simulink model "aae301_final_simulink"  (R2021a)
settings: Solver=VariableStepAuto  StartTime=0.0  StopTime=10.0  RelTol=1e-3
libraries: simulink x1
settings Model: Creator=cjobr  LastModifiedBy=cjobr

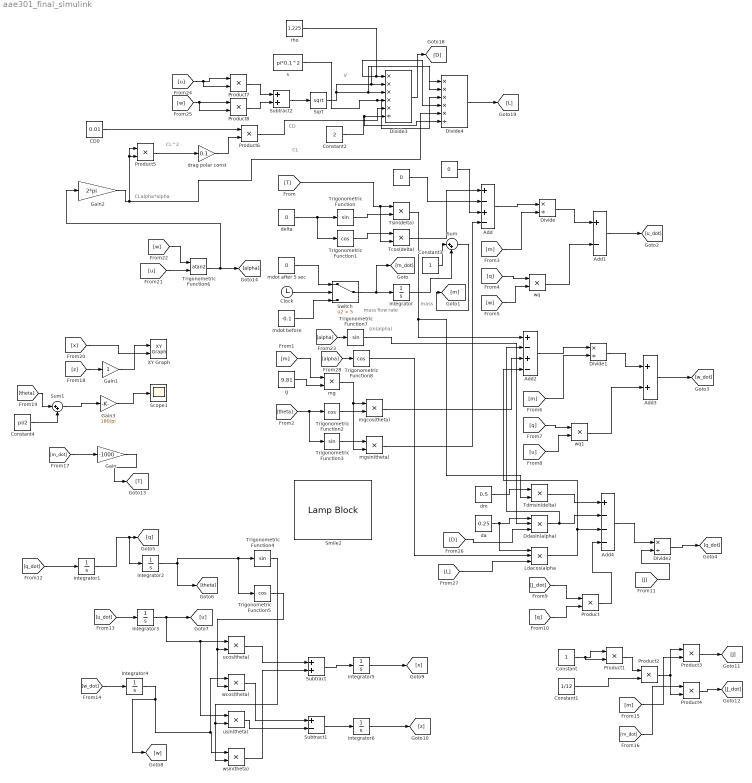
== system aae301_final_simulink ==
  note: V
  note: CL
  note: CD
  note: CL^2
  note: CLalpha*alpha
  note: sin(alpha)
  note: mass flow rate
  note: mass
  "  " : Constant  Value=0
  "    " : Constant  Value=0
  Add : Sum  Inputs=+-+-
  Add1 : Sum  Inputs=+-
  Add2 : Sum  Inputs=+-+-
  Add3 : Sum
  Add4 : Sum  Inputs=+---
  CD0 : Constant  Value=0.01
  Clock : Clock
  Constant : Constant
  Constant1 : Constant  Value=1/12
  Constant2 : Constant  Value=2
  Constant3 : Constant
  Constant4 : Constant  Value=pi/2
  Ddasin(alpha) : Product  Inputs=3
  Divide : Product  Inputs=*/
  Divide1 : Product  Inputs=*/
  Divide2 : Product  Inputs=*/
  Divide3 : Product  Inputs=*****/
  Divide4 : Product  Inputs=*****/
  Gain : Gain  Gain=-1000
  Gain1 : Gain
  Gain2 : Gain  Gain=2*pi
  Gain3 : Gain  Gain=180/pi
  Integrator{,1..6} (7 alike) : Integrator
  Ldacos(alpha : Product  Inputs=3
  Product{,1..8} (9 alike) : Product
  Scope1 : Scope
  Smile2 : LampBlock  LabelPosition=Hide  Icon=Smile2
  Sqrt : Sqrt  SaturateOnIntegerOverflow=on
  Subtract : Sum
  Subtract1 : Sum  Inputs=+-
  Subtract2 : Sum
  Sum : Sum  Inputs=|++
  Sum1 : Sum  Inputs=|++
  Switch : Switch  Criteria=u2 > Threshold  Threshold=5
  Tcos(delta) : Product
  Tdmsin(delta) : Product
  Trigonometric Function{,3..4,7} (4 alike) : Trigonometry
  Trigonometric Function{1..2,5,8} (4 alike) : Trigonometry  Operator=cos
  Trigonometric Function6 : Trigonometry  Operator=atan2
  Tsin(delta) : Product
  XY Graph : simulink/Sinks/XY Graph  xmin=-100  xmax=1700  ymin=-10  ymax=3300  st=9
  da : Constant  Value=0.25
  delta : Constant  Value=0
  dm : Constant  Value=0.5
  drag polar const : Gain  Gain=0.1
  g : Constant  Value=9.81
  "mdot after 5 sec " : Constant  Value=0
  mdot before : Constant  Value=-0.1
  mg : Product
  mgcos(theta) : Product
  mgsin(theta) : Product
  rho : Constant  Value=1.225
  s : Constant  Value=pi*0.1^2
  ucos(theta) : Product
  usin(theta) : Product
  wcos(theta) : Product
  wq : Product
  wq1 : Product
  wsin(theta) : Product
  wires:
  "mdot after 5 sec "/1 -> Switch/1
  mdot before/1 -> Switch/3
  Clock/1 -> Switch/2
  Switch/1 -> [m_dot], Integrator/1
  delta/1 -> Trigonometric Function1/1, Trigonometric Function/1
  [T] -> Tcos(delta)/2, Tsin(delta)/1
  Trigonometric Function/1 -> Tsin(delta)/2
  Trigonometric Function1/1 -> Tcos(delta)/1
  Tcos(delta)/1 -> Add/1
  "  "/1 -> Add/2
  "    "/1 -> Add/3
  g/1 -> mg/2
  [m] -> mg/1
  [theta] -> Trigonometric Function3/1, Trigonometric Function2/1
  Trigonometric Function3/1 -> mgsin(theta)/1
  Trigonometric Function2/1 -> mgcos(theta)/2
  mg/1 -> mgsin(theta)/2, mgcos(theta)/1
  mgsin(theta)/1 -> Add/4
  Add/1 -> Divide/1
  [m] -> Divide/2
  [q] -> wq/1
  [w] -> wq/2
  Divide/1 -> Add1/1
  wq/1 -> Add1/2
  Add1/1 -> [u_dot]
  Tsin(delta)/1 -> Tdmsin(delta)/2, Add2/1
  Trigonometric Function8/1 -> Ldacos(alpha/2
  mgcos(theta)/1 -> Add2/3
  wq1/1 -> Add3/2
  [m] -> Divide1/2
  [u] -> wq1/2
  [q] -> wq1/1
  Divide1/1 -> Add3/1
  Add3/1 -> [w_dot]
  Add2/1 -> Divide1/1
  dm/1 -> Tdmsin(delta)/1
  da/1 -> Ldacos(alpha/1, Ddasin(alpha)/1
  Tdmsin(delta)/1 -> Add4/1
  Ddasin(alpha)/1 -> Add2/2, Add4/2
  Ldacos(alpha/1 -> Add2/4, Add4/3
  [J_dot] -> Product/1
  [q] -> Product/2
  Product/1 -> Add4/4
  [J] -> Divide2/2
  Add4/1 -> Divide2/1
  Divide2/1 -> [q_dot]
  [q_dot] -> Integrator1/1
  Integrator1/1 -> Integrator2/1, [q]
  Integrator2/1 -> [theta], Trigonometric Function5/1, Trigonometric Function4/1
  [u_dot] -> Integrator3/1
  Integrator3/1 -> usin(theta)/1, ucos(theta)/1, [u]
  Trigonometric Function5/1 -> wcos(theta)/2, ucos(theta)/2
  Trigonometric Function4/1 -> wsin(theta)/2, usin(theta)/2
  [w_dot] -> Integrator4/1
  Integrator4/1 -> wcos(theta)/1, wsin(theta)/1, [w]
  ucos(theta)/1 -> Subtract/1
  wsin(theta)/1 -> Subtract/2
  wcos(theta)/1 -> Subtract1/1
  usin(theta)/1 -> Subtract1/2
  Subtract1/1 -> Integrator6/1
  Subtract/1 -> Integrator5/1
  Integrator5/1 -> [x]
  Integrator6/1 -> [z]
  Constant/1 -> Product1/2, Product1/1
  Constant1/1 -> Product2/2
  Product1/1 -> Product2/1
  Product2/1 -> Product4/2, Product3/1
  [m] -> Product3/2
  [m_dot] -> Product4/1
  Product4/1 -> [J_dot]
  Product3/1 -> [J]
  [m_dot] -> Gain/1
  Gain/1 -> [T]
  [z] -> Gain1/1
  [x] -> XY Graph/2
  Gain1/1 -> XY Graph/1
  [theta] -> Sum1/1
  [w] -> Trigonometric Function6/1
  [u] -> Trigonometric Function6/2
  Trigonometric Function6/1 -> Gain2/1, [alpha]
  [alpha] -> Trigonometric Function7/1
  Gain2/1 -> Divide4/5, Product5/2, Product5/1
  Product5/1 -> drag polar const/1
  CD0/1 -> Product6/1
  drag polar const/1 -> Product6/2
  Product6/1 -> Divide3/5
  [w] -> Product8/2, Product8/1
  [u] -> Product7/2, Product7/1
  Subtract2/1 -> Sqrt/1
  Product7/1 -> Subtract2/1
  Product8/1 -> Subtract2/2
  Sqrt/1 -> Divide3/2, Divide4/1, Divide3/3, Divide4/2
  rho/1 -> Divide3/1, Divide4/4
  s/1 -> Divide4/3, Divide3/4
  Constant2/1 -> Divide3/6, Divide4/6
  Divide3/1 -> [D]
  Divide4/1 -> [L]
  [D] -> Ddasin(alpha)/3
  [L] -> Ldacos(alpha/3
  Trigonometric Function7/1 -> Ddasin(alpha)/2
  [alpha] -> Trigonometric Function8/1
  Constant3/1 -> Sum/1
  Integrator/1 -> Sum/2
  Sum/1 -> [m]
  Constant4/1 -> Sum1/2
  Sum1/1 -> Gain3/1
  Gain3/1 -> Scope1/1
